simulink model "DC_Motor"  (R2021a)
settings: Solver=VariableStepAuto  StartTime=0.0  StopTime=0.6  MaxStep=0.001  RelTol=1e-3
values from neighbouring files (symbols this model uses):
  Bm = 1e-08    [DCmotorPar.m]
  Jm = 2.5e-05    [DCmotorPar.m]
  Ke = 0.066    [DCmotorPar.m]
  Kt = 0.066    [DCmotorPar.m]
  La = 1600e-6    (= 0.0016)    [DCmotorPar.m]
  Ra = 4.8    [DCmotorPar.m]
libraries: pid_lib x1
settings Model: Creator=yr13236  LastModifiedBy=DaiXingRong
settings SolverCC: ZeroCrossControl=DisableAll  AlgebraicLoopSolver=TrustRegion
settings DataIOCC: ReturnWorkspaceOutputs=off
settings DebuggingCC: SFMachineParentedDataDiag=warning  ArithmeticOperatorsInVariantConditions=warning
settings SFSimCC: SimUseLocalCustomCode=off  CustomCodeUndefinedFunction=UseInterfaceOnly
settings RTWCC: RTWUseLocalCustomCode=off

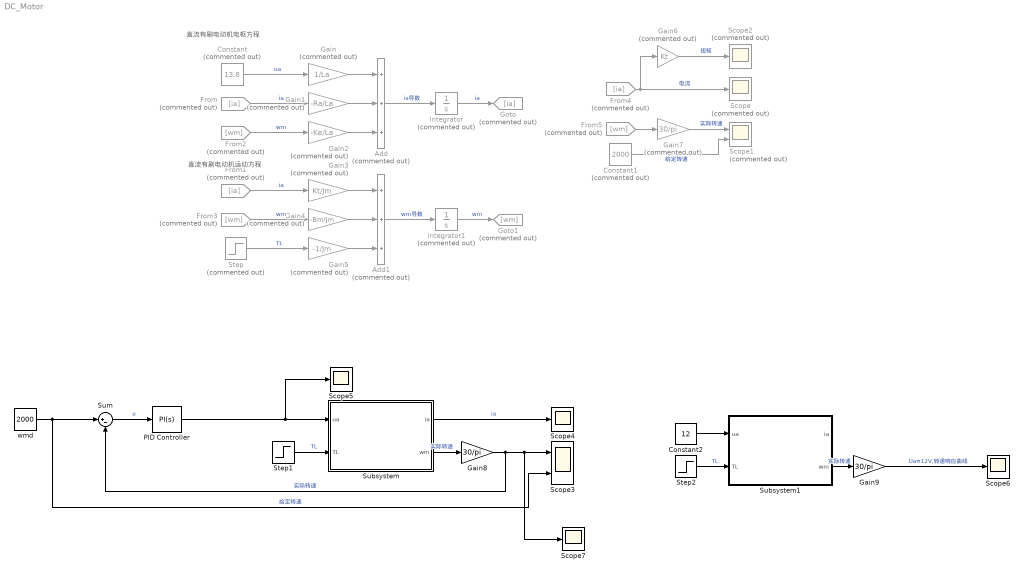
== system DC_Motor ==
  note: 直流有刷电动机运动方程
  note: 直流有刷电动机电枢方程
  Add : Sum  Commented=on  Inputs=+++
  Add1 : Sum  Commented=on  Inputs=+++
  Constant : Constant  Commented=on  Value=13.8
  Constant1 : Constant  Commented=on  Value=2000
  Constant2 : Constant  Value=12  SampleTime=0.01
  From : From  Commented=on  GotoTag=ia
  From1 : From  Commented=on  GotoTag=ia
  From2 : From  Commented=on  GotoTag=wm
  From3 : From  Commented=on  GotoTag=wm
  From4 : From  Commented=on  GotoTag=ia
  From5 : From  Commented=on  GotoTag=wm
  Gain : Gain  Commented=on  Gain=1/La
  Gain1 : Gain  Commented=on  Gain=-Ra/La
  Gain2 : Gain  Commented=on  Gain=-Ke/La
  Gain3 : Gain  Commented=on  Gain=Kt/Jm
  Gain4 : Gain  Commented=on  Gain=-Bm/Jm
  Gain5 : Gain  Commented=on  Gain=-1/Jm
  Gain6 : Gain  Commented=on  Gain=Kt
  Gain7 : Gain  Commented=on  Gain=30/pi
  Gain8 : Gain  Gain=30/pi
  Gain9 : Gain  Gain=30/pi
  Goto : Goto  Commented=on  GotoTag=ia
  Goto1 : Goto  Commented=on  GotoTag=wm
  Integrator : Integrator  Commented=on
  Integrator1 : Integrator  Commented=on
  PID Controller : pid_lib/PID Controller  Controller=PI  Form=Parallel  TimeDomain=Continuous-time  UseExternalTs=off  SampleTime=-1  IntegratorMethod=Forward Euler  FilterMethod=Forward Euler  ControllerParametersSource=internal  P=0.1  I=3  D=0  UseFilter=on  N=100  TunerSelectOption=Transfer Function Based (PID Tuner App)  InitialConditionSource=internal  InitialConditionForIntegrator=0  InitialConditionForFilter=0  DifferentiatorICPrevScaledInput=0  ExternalReset=none  TrackingMode=off  Kt=1  LimitOutput=off  SatLimitsSource=internal  UpperSaturationLimit=24  LowerSaturationLimit=-24  LinearizeAsGain=on  AntiWindupMode=back-calculation  Kb=50  POutMin=[]  POutMax=[]  IOutMin=[]  IOutMax=[]  DOutMin=[]  DOutMax=[]  NOutMin=[]  NOutMax=[]  SumOutMin=[]  SumOutMax=[]  SaturationOutMin=[]  SaturationOutMax=[]  PParamMin=[]  PParamMax=[]  IParamMin=[]  IParamMax=[]  DParamMin=[]  DParamMax=[]  NParamMin=[]  NParamMax=[]  KbParamMin=[]  KbParamMax=[]  KtParamMin=[]  KtParamMax=[]  KbOutMin=[]  KbOutMax=[]  KtOutMin=[]  KtOutMax=[]  IntegratorOutMin=[]  IntegratorOutMax=[]  FilterOutMin=[]  FilterOutMax=[]  SumI1OutMin=[]  SumI1OutMax=[]  SumI2OutMin=[]  SumI2OutMax=[]  SumI3OutMin=[]  SumI3OutMax=[]  SumI4OutMin=[]  SumI4OutMax=[]  SumDOutMin=[]  SumDOutMax=[]  DifferentiatorOutMin=[]  DifferentiatorOutMax=[]  FilterDiffOutCoefMin=[]  FilterDiffOutCoefMax=[]  ReciprocalOutMin=[]  ReciprocalOutMax=[]  SumDenOutMin=[]  SumDenOutMax=[]  SumNumOutMin=[]  SumNumOutMax=[]  DivideOutMin=[]  DivideOutMax=[]  UdiffTsProdOutMin=[]  UdiffTsProdOutMax=[]  NTsProdOutMin=[]  NTsProdOutMax=[]  UintegralTsProdOutMin=[]  UintegralTsProdOutMax=[]  UngainTsProdOutMin=[]  UngainTsProdOutMax=[]  IntegratorContinuousStateAttributes=''  IntegratorStateMustResolveToSignalObject=off  IntegratorRTWStateStorageClass=Auto  FilterContinuousStateAttributes=''  FilterStateMustResolveToSignalObject=off  FilterRTWStateStorageClass=Auto  ParallelPVariant=InternalParameters  IdealPVariant=Disabled  IVariant=InternalParameters  DVariant=Disabled  IntegratorVariant=Continuous  SatVariant=Disabled  AWVariant=Passthrough  PCopyVariant=Disabled  TRVariant=Disabled  FdbkBlocksVariant=Forward  IdealPFdbkVariant=Disabled  SatFdbkVariant=Disabled  DerivativeFilterVariant=Disabled  NVariant=Disabled  NCopyVariant=Disabled_SignalSpec  FilterICVariant=Disabled  IntegratorICVariant=InternalICs  ExternalResetVariant=Disabled  TRSumVariant=Passthrough  SumFdbkVariant=Disabled  SumVariant=Sum_PI  TsampFilterVariant=InternalTs  TsampNgainVariant=Passthrough  TsampIntegralVariant=Passthrough  ExternalSaturationOutDataTypeStr=Inherit: Same as second input
  Scope : Scope  Commented=on
  Scope1 : Scope  Commented=on  NumInputPorts=2
  Scope2 : Scope  Commented=on
  Scope3 : Scope  NumInputPorts=2
  Scope{4..7} (4 alike) : Scope
  Step : Step  Commented=on  Time=0.5  After=0.05  SampleTime=0
  Step1 : Step  Time=0.3  SampleTime=0
  Step2 : Step  Time=0.5  After=0  SampleTime=0
  Subsystem : Subsystem  mask{Ra=4.8, La=1600e-6, Ke=0.066, Kt=0.066, Jm=2.5e-05, Bm=1e-8}
      mask prompts: Ra "电阻Ra"; La "电感La"; Ke "反电动势系数Ke"; Kt "扭矩系数Kt"; Jm "转动惯量Jm"; Bm "粘性摩擦系数Bm"
      mask Display: disp('直流有刷Motor')
  Subsystem1 : Subsystem  mask{Ra=4.8, La=1600e-6, Ke=0.066, Kt=0.066, Jm=2.5e-05, Bm=1e-8}
      mask prompts: Ra "电阻Ra"; La "电感La"; Ke "反电动势系数Ke"; Kt "扭矩系数Kt"; Jm "转动惯量Jm"; Bm "粘性摩擦系数Bm"
      mask Display: disp('直流有刷Motor')
  Sum : Sum  Inputs=|+-
  wmd : Constant  Value=2000
  wires:
  Integrator/1 -> Goto/1  "ia"
  Add/1 -> Integrator/1  "ia导数"
  Integrator1/1 -> Goto1/1  "wm"
  Add1/1 -> Integrator1/1  "wm导数"
  Gain/1 -> Add/1
  Constant/1 -> Gain/1  "ua"
  Gain1/1 -> Add/2
  Gain2/1 -> Add/3
  From2/1 -> Gain2/1  "wm"
  From/1 -> Gain1/1  "ia"
  Gain4/1 -> Add1/2
  From3/1 -> Gain4/1  "wm"
  Step/1 -> Gain5/1  "TL"
  Gain5/1 -> Add1/3
  Gain3/1 -> Add1/1
  From1/1 -> Gain3/1  "ia"
  From4/1 -> Gain6/1, Scope/1  "电流"
  From5/1 -> Gain7/1
  Gain6/1 -> Scope2/1  "扭矩"
  Gain7/1 -> Scope1/1  "实际转速"
  Constant1/1 -> Scope1/2  "给定转速"
  Step1/1 -> Subsystem/2(TL)  "TL"
  wmd/1 -> Scope3/2, Sum/1  "给定转速"
  Subsystem/2(wm) -> Gain8/1  "实际转速"
  Sum/1 -> PID Controller/1  "e"
  Subsystem/1(ia) -> Scope4/1  "ia"
  Gain8/1 -> Sum/2, Scope7/1, Scope3/1  "实际转速"
  PID Controller/1 -> Scope5/1, Subsystem/1(ua)
  Constant2/1 -> Subsystem1/1(ua)
  Step2/1 -> Subsystem1/2(TL)  "TL"
  Subsystem1/2(wm) -> Gain9/1  "实际转速"
  Gain9/1 -> Scope6/1  "Ua=12V,转速响应曲线"

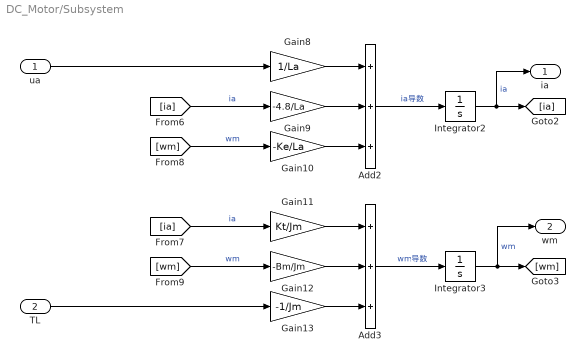
== system DC_Motor/Subsystem ==
  ua : Inport
  TL : Inport  Port=2
  Add2 : Sum  Inputs=+++
  Add3 : Sum  Inputs=+++
  Gain10 : Gain  Gain=-Ke/La
  Gain11 : Gain  Gain=Kt/Jm
  Gain12 : Gain  Gain=-Bm/Jm
  Gain13 : Gain  Gain=-1/Jm
  Gain8 : Gain  Gain=1/La
  Gain9 : Gain  Gain=-4.8/La
  Integrator2 : Integrator
  Integrator3 : Integrator
  ia : Outport  VectorParamsAs1DForOutWhenUnconnected=off
  wm : Outport  Port=2  VectorParamsAs1DForOutWhenUnconnected=off
  wires:
  [wm] -> Gain12/1  "wm"
  Gain10/1 -> Add2/3
  [wm] -> Gain10/1  "wm"
  Gain8/1 -> Add2/1
  Add2/1 -> Integrator2/1  "ia导数"
  Integrator2/1 -> ia/1, [ia]  "ia"
  Gain9/1 -> Add2/2
  [ia] -> Gain9/1  "ia"
  [ia] -> Gain11/1  "ia"
  Gain12/1 -> Add3/2
  Add3/1 -> Integrator3/1  "wm导数"
  Integrator3/1 -> wm/1, [wm]  "wm"
  ua/1 -> Gain8/1
  Gain11/1 -> Add3/1
  TL/1 -> Gain13/1
  Gain13/1 -> Add3/3

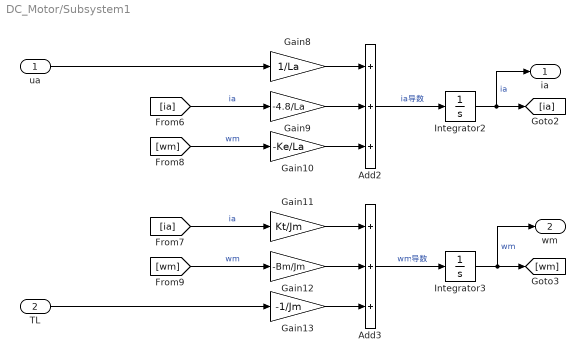
== system DC_Motor/Subsystem1 ==
  ua : Inport
  TL : Inport  Port=2
  Add2 : Sum  Inputs=+++
  Add3 : Sum  Inputs=+++
  Gain10 : Gain  Gain=-Ke/La
  Gain11 : Gain  Gain=Kt/Jm
  Gain12 : Gain  Gain=-Bm/Jm
  Gain13 : Gain  Gain=-1/Jm
  Gain8 : Gain  Gain=1/La
  Gain9 : Gain  Gain=-4.8/La
  Integrator2 : Integrator
  Integrator3 : Integrator
  ia : Outport  VectorParamsAs1DForOutWhenUnconnected=off
  wm : Outport  Port=2  VectorParamsAs1DForOutWhenUnconnected=off
  wires:
  [wm] -> Gain12/1  "wm"
  Gain10/1 -> Add2/3
  [wm] -> Gain10/1  "wm"
  Gain8/1 -> Add2/1
  Add2/1 -> Integrator2/1  "ia导数"
  Integrator2/1 -> ia/1, [ia]  "ia"
  Gain9/1 -> Add2/2
  [ia] -> Gain9/1  "ia"
  [ia] -> Gain11/1  "ia"
  Gain12/1 -> Add3/2
  Add3/1 -> Integrator3/1  "wm导数"
  Integrator3/1 -> wm/1, [wm]  "wm"
  ua/1 -> Gain8/1
  Gain11/1 -> Add3/1
  TL/1 -> Gain13/1
  Gain13/1 -> Add3/3
